simulink model "reference_generator"  (R2022b)
settings: Solver=VariableStepAuto  StartTime=0.0  StopTime=10  MaxStep=0.01  RelTol=1e-3
settings Model: Creator=simon  LastModifiedBy=fiala

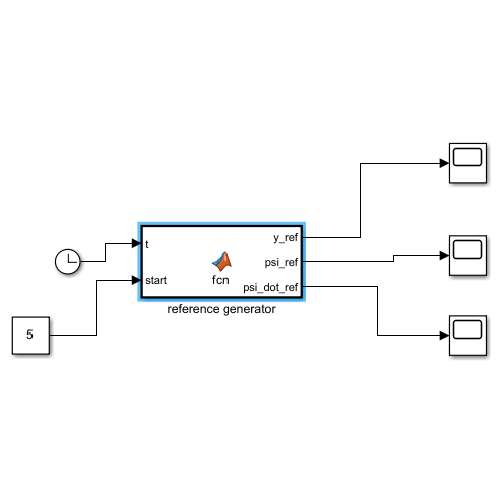
[thumbnail: Simulink's stored preview of the top-level diagram]
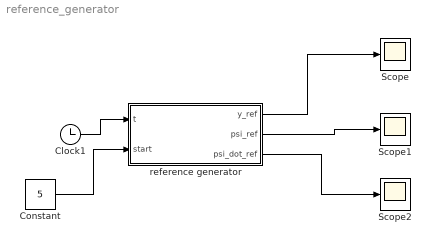
== system reference_generator ==
  Clock1 : Clock
      settings: Decimation=1000
  Constant : Constant  Value=5
  Scope : Scope
  Scope1 : Scope
  Scope2 : Scope
  reference generator : MATLAB Function  TreatAsAtomicUnit=on
  wires:
  Clock1/1 -> reference generator/1(t)
  reference generator/1(y_ref) -> Scope/1
  reference generator/2(psi_ref) -> Scope1/1
  reference generator/3(psi_dot_ref) -> Scope2/1
  Constant/1 -> reference generator/2(start)

== matlab function reference_generator/reference generator ==
  data: t input; y_ref output; psi_ref output; psi_dot_ref output; start input
function [y_ref, psi_ref, psi_dot_ref] = fcn(t, start)
    if t < start
        y_ref = 0;
        psi_ref = 0;
        psi_dot_ref = 0;
    else
        % Define the parameters
        B = 2.5; % Example value
        x1 = 30; % Example value
        y1 = 0.92; % Example value
        y_tol = 1e-7; % Example value
        C1 = log((B/y_tol) - 1);
        C2 = 5; % Example value
        Vx = 90 / 3.6;
    
        % Calculate k1, k2, k3
        k1 = (B * x1)^2 / 16 - (B * C2)^2 / 16;
        k2 = -B^2 * x1 * C1 / 8 - B * y1 * x1 + B^2 * x1 / 4;
        k3 = (B * C1)^2 / 16 + y1^2 + B^2 / 4 + B * y1 * C1 - B * y1 - B^2 * C1 / 4 - C2^2;
    
        % Calculate a and c
        a = (-k2 + sqrt(k2^2 - 4 * k1 * k3)) / (2 * k1);
        c = C1 / a;
    
        % Define the range of x
        x = Vx * (t-start);
    
        % Compute y_ref
        y_ref = B ./ (1 + exp(-a * (x - c)));
    
        % Compute the first derivative of y_ref with respect to x
    %     dydx = gradient(y_ref, x);
        dydx = (B*a*exp(a*(c - x)))/(exp(a*(c - x)) + 1)^2;
    
    
        % Compute the second derivative of y_ref with respect to x
    %     d2ydx2 = gradient(dydx, x);
        d2ydx2 = (2*B*a^2*exp(2*a*(c - x)))/(exp(a*(c - x)) + 1)^3 ...
            - (B*a^2*exp(a*(c - x)))/(exp(a*(c - x)) + 1)^2;
    
        % Define the expression for kappa_1
        kappa_1 = d2ydx2 ./ (1 + dydx.^2).^(3/2);
    
        % Compute psi_ref
        psi_ref = atan(dydx);
    
        % Compute psi_dot_ref
        psi_dot_ref = kappa_1 * Vx;
    end
end
